simulink model "fir_design"  (R2013a)
settings: Solver=ode3  StartTime=0.0  StopTime=0.1  FixedStep=1e-7  RelTol=1e-10
libraries: dspsrcs4 x2, dsparch4 x1
settings Model: Creator=admin  LastModifiedBy=admin

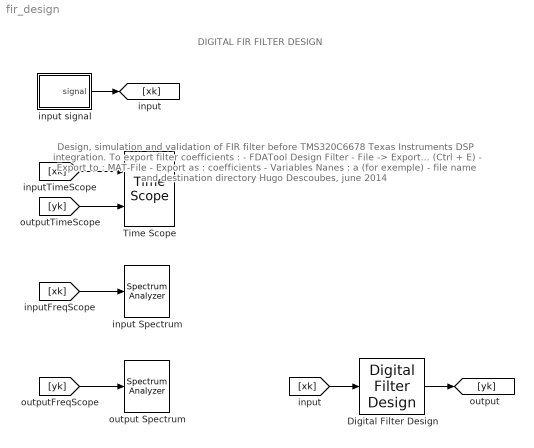
== system fir_design ==
  note: Design, simulation and validation of FIR filter before
      | TMS320C6678 Texas Instruments DSP integration.
      |
      | To export filter coefficients :
      |
      | - FDATool Design Filter
      | - File -> Export... (Ctrl + E)
      | - Export to : MAT-File
      | - Export as : coefficients
      | - Variables Nanes : a (for exemple)
      | - file name and destination directory
      |
      | Hugo Descoubes, june 2014
  note: DIGITAL FIR FILTER DESIGN
  Digital Filter Design : dsparch4/Digital Filter Design  mwdsp_browser_bugfix_var=off
  Time Scope : TimeScope  NumInputPorts=2  DefaultConfigurationName=spbscopes.TimeScopeBlockCfg
      settings: CopyFcn=scopeextensions.ScopeBlock.callback(gcbh, 'onBlockCopy', gcbh);  DeleteFcn=scopeextensions.ScopeBlock.callback(gcbh, 'onBlockDelete');  PreSaveFcn=scopeextensions.ScopeBlock.callback(gcbh, 'onModelSave');  NameChangeFcn=scopeextensions.ScopeBlock.callback(gcbh, 'onBlockRename');  CloseFcn=scopeextensions.ScopeBlock.callback(gcbh, 'onBlockClose');  PreDeleteFcn=scopeextensions.ScopeBlock.callback(gcbh, 'onBlockPreDelete');
  input Spectrum : SpectrumAnalyzer
      settings: CopyFcn=scopeextensions.ScopeBlock.callback(gcbh, 'onBlockCopy', gcbh);  DeleteFcn=scopeextensions.ScopeBlock.callback(gcbh, 'onBlockDelete');  PreSaveFcn=scopeextensions.ScopeBlock.callback(gcbh, 'onModelSave');  NameChangeFcn=scopeextensions.ScopeBlock.callback(gcbh, 'onBlockRename');  CloseFcn=scopeextensions.ScopeBlock.callback(gcbh, 'onBlockClose');  PreDeleteFcn=scopeextensions.ScopeBlock.callback(gcbh, 'onBlockPreDelete');
  input signal : Subsystem
  output Spectrum : SpectrumAnalyzer
      settings: CopyFcn=scopeextensions.ScopeBlock.callback(gcbh, 'onBlockCopy', gcbh);  DeleteFcn=scopeextensions.ScopeBlock.callback(gcbh, 'onBlockDelete');  PreSaveFcn=scopeextensions.ScopeBlock.callback(gcbh, 'onModelSave');  NameChangeFcn=scopeextensions.ScopeBlock.callback(gcbh, 'onBlockRename');  CloseFcn=scopeextensions.ScopeBlock.callback(gcbh, 'onBlockClose');  PreDeleteFcn=scopeextensions.ScopeBlock.callback(gcbh, 'onBlockPreDelete');
  wires:
  input signal/1(signal) -> [xk]
  [xk] -> Time Scope/1
  [yk] -> Time Scope/2
  [xk] -> input Spectrum/1
  [yk] -> output Spectrum/1
  [xk] -> Digital Filter Design/1
  Digital Filter Design/1 -> [yk]

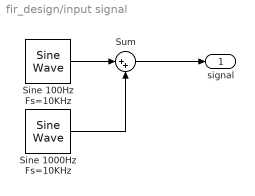
== system fir_design/input signal ==
  Sine 1000Hz Fs=10KHz : dspsrcs4/Sine Wave  Amplitude=1  Frequency=1000  Phase=0  SampleMode=Discrete  OutComplex=Real  CompMethod=Trigonometric fcn  TableSize=Speed  SampleTime=1e-4  SamplesPerFrame=1  ResetState=Restart at time zero  dataType=double  wordLen=16  udDataType=sfix(16)  fracBitsMode=Best precision  numFracBits=15  OutDataTypeStr=double  LastOutDataTypeStr=double
  Sine 100Hz Fs=10KHz : dspsrcs4/Sine Wave  Amplitude=1  Frequency=100  Phase=0  SampleMode=Discrete  OutComplex=Real  CompMethod=Trigonometric fcn  TableSize=Speed  SampleTime=1e-4  SamplesPerFrame=1  ResetState=Restart at time zero  dataType=double  wordLen=16  udDataType=sfix(16)  fracBitsMode=Best precision  numFracBits=15  OutDataTypeStr=double  LastOutDataTypeStr=double
  Sum : Sum  Inputs=|++
  signal : Outport
  wires:
  Sum/1 -> signal/1
  Sine 100Hz Fs=10KHz/1 -> Sum/1
  Sine 1000Hz Fs=10KHz/1 -> Sum/2
